simulink model "Vt"  (R2022b)
settings: Solver=FixedStepAuto  StartTime=0.0  StopTime=10.0  RelTol=1e-3
settings Model: Creator=86134  LastModifiedBy=86134

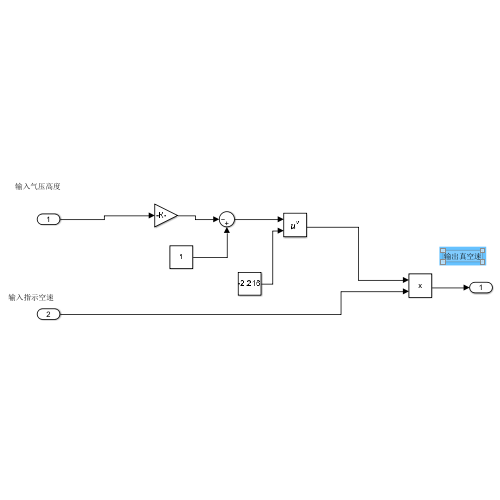
[thumbnail: Simulink's stored preview of the top-level diagram]
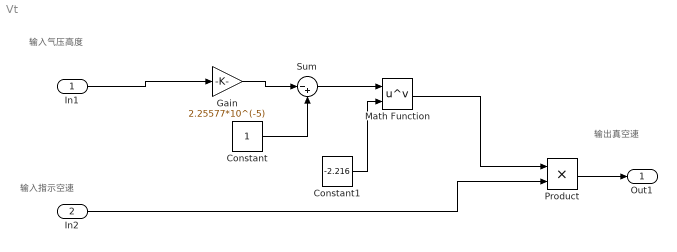
== system Vt ==
  note: 输出真空速
  note: 输入指示空速
  note: 输入气压高度
  In1 : Inport
  In2 : Inport  Port=2
  Constant : Constant
  Constant1 : Constant  Value=-2.216
  Gain : Gain  Gain=2.25577*10^(-5)
  Math Function : Math  Operator=pow
  Product : Product
  Sum : Sum  Inputs=|-+
  Out1 : Outport
  wires:
  In1/1 -> Gain/1
  Gain/1 -> Sum/1
  Constant/1 -> Sum/2
  Sum/1 -> Math Function/1
  Constant1/1 -> Math Function/2
  Math Function/1 -> Product/1
  In2/1 -> Product/2
  Product/1 -> Out1/1
